simulink model "sschdlexSolarInverterSingleNetworkExample"  (R2023b)
settings: Solver=ode23t  StartTime=0.0  StopTime=.5  MaxStep=1e-4  RelTol=1e-3
PreLoadFcn:
  | load('EmulatedPV_LowPowerData.mat');
  | irr = 0.15;
  | numIrr = 10;
  | ArrayPower = ArrayCurrent.*ArrayVoltage;
  | 
  | C_Boost_In = 680e-6;
  | C_Boost_In_R = 0;
  | L_Boost = 100e-6;
  | L_Boost_R = 0;
  | C_Boost_Out = 1640e-6;
  | 
  | TsFPGA = 2e-6;
  | TsControl = 2e-6;
  | TsCPU = 2e-6;
  | Tc = TsControl;
  | Ts = 2e-6;
  | 
  | IGBT_Vth = 6;
  | IGBT_Vf = 0.8;
  | IGBT_R = 0.001;
  | IGBT_Con = 1e-5;
  | 
  | IGBT_D_Vth = 0.8;
  | IGBT_D_R = 0.001;
  | IGBT_D_Con = 1e-5;
  | 
  | maxIn = 10;
  | minIn = -10;
  | maxOut = 2^15;
  | minOut = -2^15;
  | difIn = maxIn-minIn;
  | difOut = maxOut-minOut;
  | gain = difOut/difIn;
  | dc1 = (maxOut+minOut)/2;
  | dc2 = (maxIn+minIn)/2;
  | offset = dc1-gain*dc2;
  | numIrr = 10;
  | ArrayPower = ArrayCurrent.*ArrayVoltage;
InitFcn:
  | Ts = 2e-6;
  | Tc = Ts;
values from neighbouring files (symbols this model uses):
  ArrayCurrent = [3 2.90135967378 2.78442846347 2.64406556825 2.47269969012 2.25842875672 1.98100825201 1.60223040661 1.04533074246 0.222841716608 0 0 ... (1000 elements, 100x10)]    [EmulatedPV_LowPowerData.mat]
  ArrayVoltage = [0 0.151515151515 0.30303030303 0.454545454545 0.606060606061 0.757575757576 0.909090909091 1.06060606061 1.21212121212 1.36363636364 1.51515151515 1.66666666667 ... (100 elements, 100x1)]    [EmulatedPV_LowPowerData.mat]
  Irradiance = [0.05 0.1 0.15 0.2 0.25 0.3 0.35 0.4 0.45 0.5]    [EmulatedPV_LowPowerData.mat]
undefined symbols (not defined in the file or in its folder): DiscIntNeverNeededParam, Tdata
libraries: fl_lib x20, nesl_utility x12, ee_lib x5, powerlib_meascontrol x4, simulink x3, slpidlib x2
CloseFcn:
  | clear ArrayCurrent
  | clear ArrayVoltage
  | clear Irradiance
  | 
  | clear irr;
  | clear numIrr;
  | clear ArrayPower;
  | 
  | clear C_Boost_In;
  | clear C_Boost_In_R;
  | clear L_Boost;
  | clear L_Boost_R;
  | clear C_Boost_Out;
  | 
  | clear TsFPGA;
  | clear TsControl;
  | clear TsCPU;
  | clear Tc;
  | clear Ts;
  | 
  | clear IGBT_Vth;
  | clear IGBT_Vf;
  | clear IGBT_R ;
  | clear IGBT_Con;
  | 
  | clear IGBT_D_Vth;
  | clear IGBT_D_R;
  | clear IGBT_D_Con;
  | 
  | clear maxIn;
  | clear minIn;
  | clear maxOut;
  | clear minOut;
  | clear difIn;
  | clear difOut;
  | clear gain;
  | clear dc1;
  | clear dc2;
  | clear offset;
settings Model: Creator=The MathWorks, Inc.  LastModifiedBy=The MathWorks, Inc.
settings SolverCC: AlgebraicLoopSolver=TrustRegion  AutoInsertRateTranBlk=on
settings OptimizationCC: BlockReduction=off  ConditionallyExecuteInputs=off  DefaultParameterBehavior=Inlined  EfficientMapNaN2IntZero=off
settings DebuggingCC: AlgebraicLoopMsg=error  SingleTaskRateTransMsg=error  ParameterPrecisionLossMsg=none  UnconnectedInputMsg=warning  UnconnectedOutputMsg=warning  UnconnectedLineMsg=warning  PregeneratedLibrarySubsystemCodeDiagnostic=none  ArithmeticOperatorsInVariantConditions=warning
settings HardwareCC: ProdBitPerPointer=32  ProdBitPerSizeT=32  ProdBitPerPtrDiffT=32  ProdLargestAtomicFloat=None  ProdIntDivRoundTo=Undefined  ProdEndianess=Unspecified  ProdWordSize=32  ProdHWDeviceType=ASIC/FPGA->ASIC/FPGA  TargetBitPerPointer=64  TargetBitPerSizeT=64  TargetBitPerPtrDiffT=64  TargetLongLongMode=on  TargetIntDivRoundTo=Zero  TargetEndianess=LittleEndian  TargetWordSize=64  TargetHWDeviceType=Custom Processor->MATLAB Host Computer  ProdEqTarget=off
settings ModelReferenceCC: EnableRefExpFcnMdlSchedulingChecks=on
settings SFSimCC: SimUseLocalCustomCode=off
settings CodeAppCC: MaxIdLength=128
settings GRTTargetCC: TargetLangStandard=C89/C90 (ANSI)  CombineOutputUpdateFcns=off  GRTInterface=on

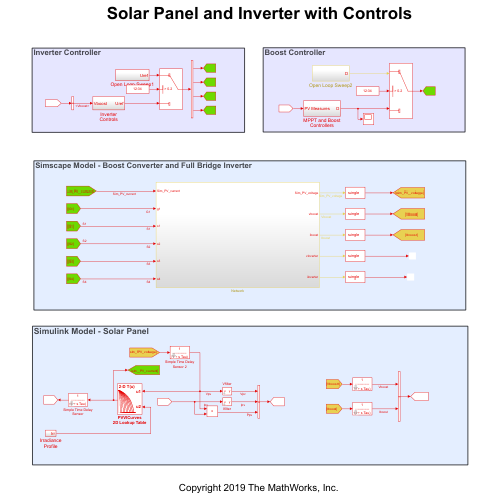
[thumbnail: Simulink's stored preview of the top-level diagram]
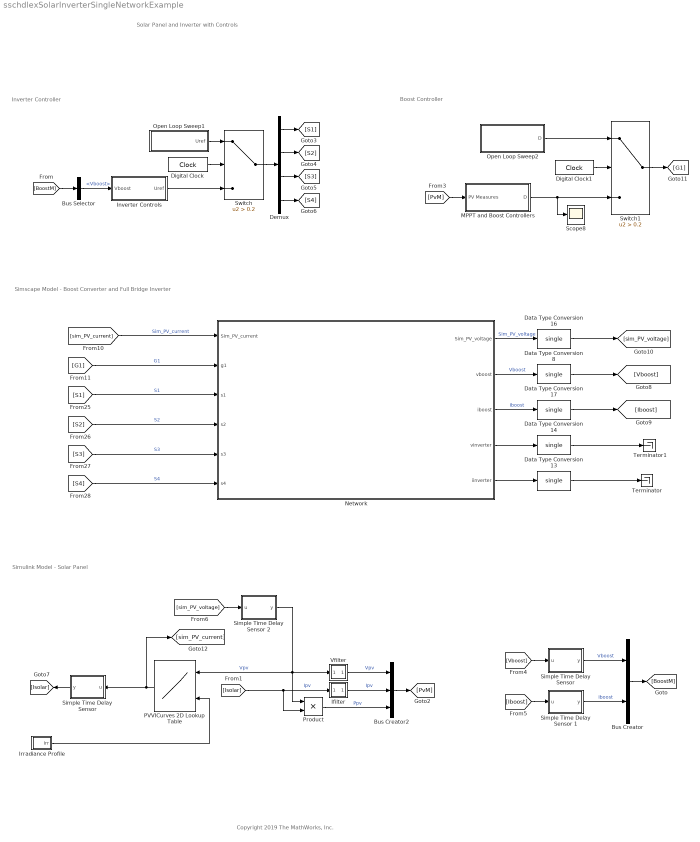
== system sschdlexSolarInverterSingleNetworkExample ==
  note: Solar Panel and Inverter with Controls
  note: Simulink Model - Solar Panel
  note: Inverter Controller
  note: Boost Controller
  note: Simscape Model - Boost Converter and Full Bridge Inverter
  note: Copyright 2019 The MathWorks, Inc.
  Bus Creator : BusCreator  Inputs=2
  Bus Creator2 : BusCreator  Inputs=3
  Bus Selector : BusSelector  OutputSignals=Vboost
  Data Type Conversion{13..14,16..17} (4 alike) : DataTypeConversion  OutDataTypeStr=single  RndMeth=Nearest  SaturateOnIntegerOverflow=off
  Data Type Conversion8 : DataTypeConversion  OutDataTypeStr=single  SaturateOnIntegerOverflow=off  RndMeth=Floor
  Demux : Demux
  Digital Clock : DigitalClock  SampleTime=2e-6
  Digital Clock1 : DigitalClock  SampleTime=2e-6
  Ifilter : Subsystem  mask{Tf=0.01}
      mask prompts: Tf "Filter Time Constant"
  Inverter Controls : Subsystem
  Irradiance Profile : Subsystem
  MPPT and Boost Controllers : Subsystem
  Network : Subsystem
  Open Loop Sweep1 : Subsystem
  Open Loop Sweep2 : Subsystem
  PVVICurves 2D Lookup Table : Lookup_n-D  BreakpointsForDimension1=ArrayVoltage  BreakpointsForDimension2=Irradiance  Table=ArrayCurrent  InternalRulePriority=Speed  RndMeth=Simplest
      settings: InputPortMap=u0,u1
  Product : Product
  Scope8 : Scope
  Simple Time Delay Sensor : Subsystem  mask{Ts=Ts, Tau=0.0001}
      mask prompts: Ts "Sample Time, [s]"; Tau "Time Constant, Tau [s]"
      mask help: Simple Sensor
      mask Display: fprintf('1\n------------\n(1 + s Tau)');
  "Simple Time Delay Sensor " : Subsystem  mask{Ts=Ts, Tau=0.0001}
      mask prompts: Ts "Sample Time, [s]"; Tau "Time Constant, Tau [s]"
      mask help: Simple Sensor
      mask Display: fprintf('1\n------------\n(1 + s Tau)');
  Simple Time Delay Sensor 1 : Subsystem  mask{Ts=Ts, Tau=0.0001}
      mask prompts: Ts "Sample Time, [s]"; Tau "Time Constant, Tau [s]"
      mask help: Simple Sensor
      mask Display: fprintf('1\n------------\n(1 + s Tau)');
  Simple Time Delay Sensor 2 : Subsystem  mask{Ts=Ts, Tau=0.0001}
      mask prompts: Ts "Sample Time, [s]"; Tau "Time Constant, Tau [s]"
      mask help: Simple Sensor
      mask Display: fprintf('1\n------------\n(1 + s Tau)');
  Switch : Switch  Criteria=u2 > Threshold  Threshold=0.2  SaturateOnIntegerOverflow=off  InputSameDT=off
  Switch1 : Switch  Criteria=u2 > Threshold  Threshold=0.2  SaturateOnIntegerOverflow=off  InputSameDT=off
  Terminator : Terminator
  Terminator1 : Terminator
  Vfilter : Subsystem  mask{Tf=0.01}
      mask prompts: Tf "Filter Time Constant"
  wires:
  Bus Creator/1 -> [BoostM]
  Demux/3 -> [S3]
  Demux/2 -> [S2]
  Irradiance Profile/1(Irr) -> PVVICurves 2D Lookup Table/2
  Product/1 -> Bus Creator2/3  "Ppv"
  Vfilter/1(y) -> Bus Creator2/1  "Vpv"
  [PvM] -> MPPT and Boost Controllers/1(PV Measures)
  PVVICurves 2D Lookup Table/1 -> Simple Time Delay Sensor/1(u), [sim_PV_current]
  [sim_PV_voltage] -> Simple Time Delay Sensor 2/1(u)
  MPPT and Boost Controllers/1(D) -> Scope8/1, Switch1/3
  [Iboost] -> Simple Time Delay Sensor 1/1(u)
  Open Loop Sweep1/1(Uref) -> Switch/1
  Bus Selector/1 -> Inverter Controls/1(Vboost)  "<Vboost>"
  Digital Clock1/1 -> Switch1/2
  Ifilter/1(y) -> Bus Creator2/2  "Ipv"
  [Isolar] -> Product/2, Ifilter/1(u)  "Ipv"
  Switch/1 -> Demux/1
  Switch1/1 -> [G1]
  Simple Time Delay Sensor/1(y) -> [Isolar]
  Bus Creator2/1 -> [PvM]
  Simple Time Delay Sensor 2/1(y) -> PVVICurves 2D Lookup Table/1, Product/1, Vfilter/1(u)  "Vpv"
  Simple Time Delay Sensor 1/1(y) -> Bus Creator/2  "Iboost"
  [Vboost] -> "Simple Time Delay Sensor "/1(u)
  Demux/1 -> [S1]
  Demux/4 -> [S4]
  [BoostM] -> Bus Selector/1
  Open Loop Sweep2/1(D) -> Switch1/1
  "Simple Time Delay Sensor "/1(y) -> Bus Creator/1  "Vboost"
  Inverter Controls/1(Uref) -> Switch/3
  Digital Clock/1 -> Switch/2
  [S4] -> Network/6(s4)  "S4"
  [S2] -> Network/4(s2)  "S2"
  [S1] -> Network/3(s1)  "S1"
  Data Type Conversion8/1 -> [Vboost]
  Data Type Conversion16/1 -> [sim_PV_voltage]
  Data Type Conversion17/1 -> [Iboost]
  [sim_PV_current] -> Network/1(Sim_PV_current)  "Sim_PV_current"
  Network/1(Sim_PV_voltage) -> Data Type Conversion16/1  "Sim_PV_voltage"
  Network/3(iboost) -> Data Type Conversion17/1  "Iboost"
  Network/2(vboost) -> Data Type Conversion8/1  "Vboost"
  [G1] -> Network/2(g1)  "G1"
  Data Type Conversion13/1 -> Terminator/1
  Data Type Conversion14/1 -> Terminator1/1
  [S3] -> Network/5(s3)  "S3"
  Network/4(vinverter) -> Data Type Conversion14/1
  Network/5(iinverter) -> Data Type Conversion13/1

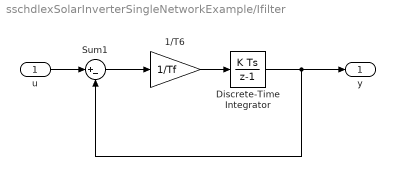
== system sschdlexSolarInverterSingleNetworkExample/Ifilter ==
  u : Inport
  1/T6 : Gain  Gain=1/Tf
  Discrete-Time Integrator : DiscreteIntegrator  SampleTime=Tc  ICPrevOutput=DiscIntNeverNeededParam  ICPrevScaledInput=DiscIntNeverNeededParam
  Sum1 : Sum  Inputs=|+-
  y : Outport  VectorParamsAs1DForOutWhenUnconnected=off
  wires:
  Sum1/1 -> 1/T6/1
  Discrete-Time Integrator/1 -> Sum1/2, y/1
  u/1 -> Sum1/1
  1/T6/1 -> Discrete-Time Integrator/1

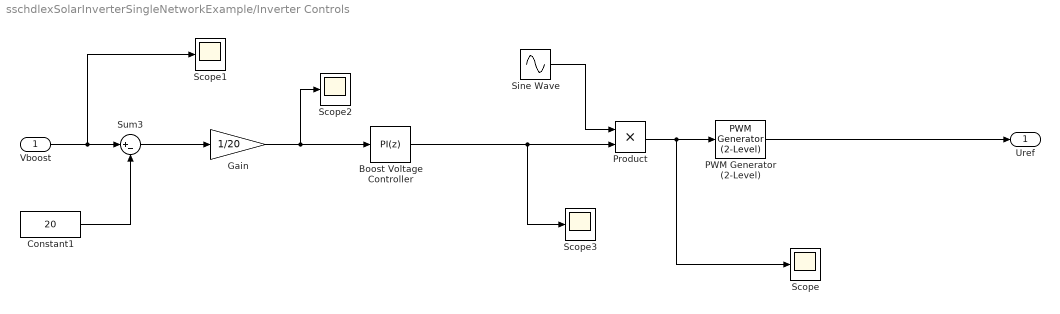
== system sschdlexSolarInverterSingleNetworkExample/Inverter Controls ==
  Vboost : Inport
  Boost Voltage Controller : slpidlib/PID Controller  Controller=PI  Form=Parallel  TimeDomain=Discrete-time  UseExternalTs=off  SampleTime=Tc  IntegratorMethod=Forward Euler  FilterMethod=Forward Euler  ControllerParametersSource=internal  P=4  I=500  UseKiTs=off  D=0  N=100  UseFilter=on  TunerSelectOption=Transfer Function Based (PID Tuner App)  InitialConditionSource=internal  InitialConditionForIntegrator=1  InitialConditionForFilter=0  DifferentiatorICPrevScaledInput=0  ExternalReset=none  TrackingMode=off  Kt=1  LimitOutput=on  SatLimitsSource=internal  UpperSaturationLimit=1  LowerSaturationLimit=0  LinearizeAsGain=on  AntiWindupMode=clamping  Kb=1  LimitIntegrator=off  UpperIntegratorSaturationLimit=inf  LowerIntegratorSaturationLimit=-inf  POutMin=[]  POutMax=[]  IOutMin=[]  IOutMax=[]  DOutMin=[]  DOutMax=[]  NOutMin=[]  NOutMax=[]  SumOutMin=[]  SumOutMax=[]  SaturationOutMin=[]  SaturationOutMax=[]  PParamMin=[]  PParamMax=[]  IParamMin=[]  IParamMax=[]  DParamMin=[]  DParamMax=[]  NParamMin=[]  NParamMax=[]  KbParamMin=[]  KbParamMax=[]  KtParamMin=[]  KtParamMax=[]  KbOutMin=[]  KbOutMax=[]  KtOutMin=[]  KtOutMax=[]  IntegratorOutMin=[]  IntegratorOutMax=[]  FilterOutMin=[]  FilterOutMax=[]  SumI1OutMin=[]  SumI1OutMax=[]  SumI2OutMin=[]  SumI2OutMax=[]  SumI3OutMin=[]  SumI3OutMax=[]  SumI4OutMin=[]  SumI4OutMax=[]  SumDOutMin=[]  SumDOutMax=[]  DifferentiatorOutMin=[]  DifferentiatorOutMax=[]  FilterDiffOutCoefMin=[]  FilterDiffOutCoefMax=[]  ReciprocalOutMin=[]  ReciprocalOutMax=[]  SumDenOutMin=[]  SumDenOutMax=[]  SumNumOutMin=[]  SumNumOutMax=[]  DivideOutMin=[]  DivideOutMax=[]  UdiffTsProdOutMin=[]  UdiffTsProdOutMax=[]  NTsProdOutMin=[]  NTsProdOutMax=[]  UintegralTsProdOutMin=[]  UintegralTsProdOutMax=[]  UngainTsProdOutMin=[]  UngainTsProdOutMax=[]  ClampingZeroOutDataTypeStr=Inherit: Inherit via back propagation  ClampingZeroOutMin=[]  ClampingZeroOutMax=[]  FilterDenConstantOutDataTypeStr=Inherit: Inherit via back propagation  FilterDenConstantOutMin=[]  FilterDenConstantOutMax=[]  PCopyOutDataTypeStr=Inherit: Inherit via back propagation  PCopyOutMin=[]  PCopyOutMax=[]  NCopyOutDataTypeStr=Inherit: Inherit via back propagation  NCopyOutMin=[]  NCopyOutMax=[]  IntegratorContinuousStateAttributes=''  IntegratorStateMustResolveToSignalObject=off  IntegratorRTWStateStorageClass=Auto  FilterContinuousStateAttributes=''  FilterStateMustResolveToSignalObject=off  FilterRTWStateStorageClass=Auto  ParallelPVariant=InternalParameters  IdealPVariant=Disabled  IVariant=InternalParameters  DVariant=Disabled  IntegratorVariant=Discrete  SatVariant=Enabled  AWVariant=DiscClampingParallel  PCopyVariant=Disabled  TRVariant=Disabled  FdbkBlocksVariant=Forward  IdealPFdbkVariant=Disabled  SatFdbkVariant=Disabled  DerivativeFilterVariant=Disabled  NVariant=Disabled  NCopyVariant=Disabled_SignalSpec  FilterICVariant=Disabled  IntegratorICVariant=InternalICs  ExternalResetVariant=Disabled  TRSumVariant=Passthrough  SumFdbkVariant=Disabled  SumVariant=Sum_PI  TsampFilterVariant=InternalTs  TsampNgainVariant=Passthrough  TsampIntegralVariant=Disabled_SignalSpec  ExternalSaturationOutDataTypeStr=Inherit: Same as second input
  Constant1 : Constant  Value=20
  Gain : Gain  Gain=1/20
  "PWM Generator (2-Level) " : powerlib_meascontrol/Pulse & Signal Generators/PWM Generator (2-Level)  ModulatorType=Single-phase full-bridge (4 pulses)  ModulatorMode=Unsynchronized  Fc=2000  Pc=90  nF=27  MinMax="[ -1  1 ]"  SamplingTechnique=Natural  ModulatingSignals=off  m=0.8  Freq=60  Phase=0  Ts=TsFPGA  ShowCarrierOutport=off
  Product : Product
  Scope{,1..3} (4 alike) : Scope
  Sine Wave : Sin  Frequency=2*pi*60  SampleTime=Tc
  Sum3 : Sum  Inputs=|+-
  Uref : Outport  VectorParamsAs1DForOutWhenUnconnected=off
  wires:
  Constant1/1 -> Sum3/2
  Sine Wave/1 -> Product/1
  Boost Voltage Controller/1 -> Scope3/1, Product/2
  Sum3/1 -> Gain/1
  Vboost/1 -> Scope1/1, Sum3/1
  Gain/1 -> Scope2/1, Boost Voltage Controller/1
  Product/1 -> Scope/1, "PWM Generator (2-Level) "/1
  "PWM Generator (2-Level) "/1 -> Uref/1

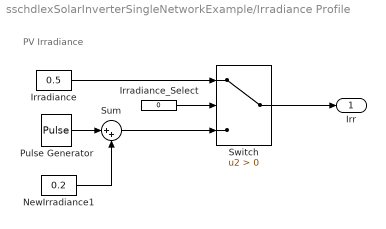
== system sschdlexSolarInverterSingleNetworkExample/Irradiance Profile ==
  note: PV Irradiance
  Irradiance : Constant  Value=0.5  OutDataTypeStr=single  SampleTime=2e-6
  Irradiance_Select : Constant  Value=0  OutDataTypeStr=single  SampleTime=2e-6
  NewIrradiance1 : Constant  Value=0.2  OutDataTypeStr=single  SampleTime=2e-6
  Pulse Generator : DiscretePulseGenerator  Amplitude=0.2  SampleTime=2e-6
  Sum : Sum  Inputs=|++
  Switch : Switch  Criteria=u2 > Threshold  SaturateOnIntegerOverflow=off  InputSameDT=off
  Irr : Outport  VectorParamsAs1DForOutWhenUnconnected=off
  wires:
  NewIrradiance1/1 -> Sum/2
  Pulse Generator/1 -> Sum/1
  Sum/1 -> Switch/3
  Irradiance/1 -> Switch/1
  Switch/1 -> Irr/1
  Irradiance_Select/1 -> Switch/2

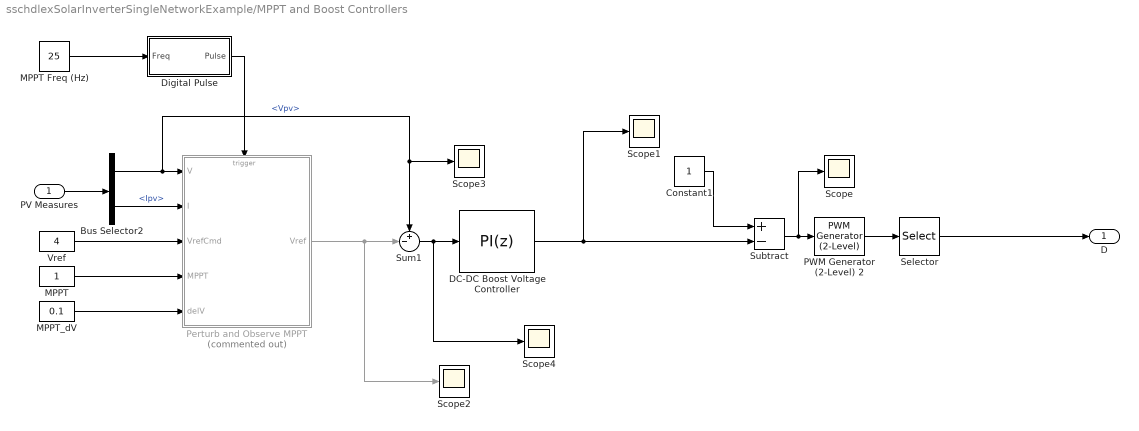
== system sschdlexSolarInverterSingleNetworkExample/MPPT and Boost Controllers ==
  PV Measures : Inport
  Bus Selector2 : BusSelector  OutputSignals=Vpv,Ipv
  Constant1 : Constant
  DC-DC Boost Voltage Controller : slpidlib/PID Controller  Controller=PI  Form=Parallel  TimeDomain=Discrete-time  UseExternalTs=off  SampleTime=Tc  IntegratorMethod=Forward Euler  FilterMethod=Forward Euler  ControllerParametersSource=internal  P=0.015  I=2.5  UseKiTs=off  D=0  N=100  UseFilter=on  TunerSelectOption=Transfer Function Based (PID Tuner App)  InitialConditionSource=internal  InitialConditionForIntegrator=0  InitialConditionForFilter=0  DifferentiatorICPrevScaledInput=0  ExternalReset=none  TrackingMode=off  Kt=1  LimitOutput=off  SatLimitsSource=internal  UpperSaturationLimit=0.9  LowerSaturationLimit=0  LinearizeAsGain=on  AntiWindupMode=clamping  Kb=1  LimitIntegrator=off  UpperIntegratorSaturationLimit=inf  LowerIntegratorSaturationLimit=-inf  POutMin=[]  POutMax=[]  IOutMin=[]  IOutMax=[]  DOutMin=[]  DOutMax=[]  NOutMin=[]  NOutMax=[]  SumOutMin=[]  SumOutMax=[]  SaturationOutMin=[]  SaturationOutMax=[]  PParamMin=[]  PParamMax=[]  IParamMin=[]  IParamMax=[]  DParamMin=[]  DParamMax=[]  NParamMin=[]  NParamMax=[]  KbParamMin=[]  KbParamMax=[]  KtParamMin=[]  KtParamMax=[]  KbOutMin=[]  KbOutMax=[]  KtOutMin=[]  KtOutMax=[]  IntegratorOutMin=[]  IntegratorOutMax=[]  FilterOutMin=[]  FilterOutMax=[]  SumI1OutMin=[]  SumI1OutMax=[]  SumI2OutMin=[]  SumI2OutMax=[]  SumI3OutMin=[]  SumI3OutMax=[]  SumI4OutMin=[]  SumI4OutMax=[]  SumDOutMin=[]  SumDOutMax=[]  DifferentiatorOutMin=[]  DifferentiatorOutMax=[]  FilterDiffOutCoefMin=[]  FilterDiffOutCoefMax=[]  ReciprocalOutMin=[]  ReciprocalOutMax=[]  SumDenOutMin=[]  SumDenOutMax=[]  SumNumOutMin=[]  SumNumOutMax=[]  DivideOutMin=[]  DivideOutMax=[]  UdiffTsProdOutMin=[]  UdiffTsProdOutMax=[]  NTsProdOutMin=[]  NTsProdOutMax=[]  UintegralTsProdOutMin=[]  UintegralTsProdOutMax=[]  UngainTsProdOutMin=[]  UngainTsProdOutMax=[]  ClampingZeroOutDataTypeStr=Inherit: Inherit via back propagation  ClampingZeroOutMin=[]  ClampingZeroOutMax=[]  FilterDenConstantOutDataTypeStr=Inherit: Inherit via back propagation  FilterDenConstantOutMin=[]  FilterDenConstantOutMax=[]  PCopyOutDataTypeStr=Inherit: Inherit via back propagation  PCopyOutMin=[]  PCopyOutMax=[]  NCopyOutDataTypeStr=Inherit: Inherit via back propagation  NCopyOutMin=[]  NCopyOutMax=[]  IntegratorContinuousStateAttributes=''  IntegratorStateMustResolveToSignalObject=off  IntegratorRTWStateStorageClass=Auto  FilterContinuousStateAttributes=''  FilterStateMustResolveToSignalObject=off  FilterRTWStateStorageClass=Auto  ParallelPVariant=InternalParameters  IdealPVariant=Disabled  IVariant=InternalParameters  DVariant=Disabled  IntegratorVariant=Discrete  SatVariant=Disabled  AWVariant=Passthrough  PCopyVariant=Disabled  TRVariant=Disabled  FdbkBlocksVariant=Forward  IdealPFdbkVariant=Disabled  SatFdbkVariant=Disabled  DerivativeFilterVariant=Disabled  NVariant=Disabled  NCopyVariant=Disabled_SignalSpec  FilterICVariant=Disabled  IntegratorICVariant=InternalICs  ExternalResetVariant=Disabled  TRSumVariant=Passthrough  SumFdbkVariant=Disabled  SumVariant=Sum_PI  TsampFilterVariant=InternalTs  TsampNgainVariant=Passthrough  TsampIntegralVariant=Disabled_SignalSpec  ExternalSaturationOutDataTypeStr=Inherit: Same as second input
  Digital Pulse : Subsystem  mask{Ts=Tc, Duty=0.5}
      mask prompts: Ts "Sample Rate [s]"; Duty "Duty Cycle [0-1]"
  MPPT : Constant
  MPPT Freq (Hz) : Constant  Value=25
  MPPT_dV : Constant  Value=0.1
  PWM Generator (2-Level) 2 : powerlib_meascontrol/Pulse & Signal Generators/PWM Generator (2-Level)  ModulatorType=Single-phase full-bridge (4 pulses)  ModulatorMode=Unsynchronized  Fc=2000  Pc=90  nF=27  MinMax=[0 1 ]  SamplingTechnique=Natural  ModulatingSignals=off  m=0.8  Freq=60  Phase=0  Ts=TsFPGA  ShowCarrierOutport=off
  Perturb and Observe MPPT : Subsystem  Commented=on  TreatAsAtomicUnit=on  SystemSampleTime=Tdata
  Scope{,1..4} (5 alike) : Scope
  Selector : Selector  InputPortWidth=4  IndexOptions=Index vector (dialog)  Indices=2  OutputSizes=1
  Subtract : Sum  Inputs=+-
  Sum1 : Sum  Inputs=+-|
  Vref : Constant  Value=4
  D : Outport  VectorParamsAs1DForOutWhenUnconnected=off
  wires:
  PV Measures/1 -> Bus Selector2/1
  Digital Pulse/1(Pulse) -> Perturb and Observe MPPT/Trigger
  MPPT Freq (Hz)/1 -> Digital Pulse/1(Freq)
  MPPT_dV/1 -> Perturb and Observe MPPT/5(delV)
  Vref/1 -> Perturb and Observe MPPT/3(VrefCmd)
  Sum1/1 -> Scope4/1, DC-DC Boost Voltage Controller/1
  MPPT/1 -> Perturb and Observe MPPT/4(MPPT)
  Bus Selector2/1 -> Perturb and Observe MPPT/1(V), Scope3/1, Sum1/1  "<Vpv>"
  Perturb and Observe MPPT/1(Vref) -> Scope2/1, Sum1/2
  Bus Selector2/2 -> Perturb and Observe MPPT/2(I)  "<Ipv>"
  Selector/1 -> D/1
  PWM Generator (2-Level) 2/1 -> Selector/1
  Constant1/1 -> Subtract/1
  DC-DC Boost Voltage Controller/1 -> Scope1/1, Subtract/2
  Subtract/1 -> Scope/1, PWM Generator (2-Level) 2/1

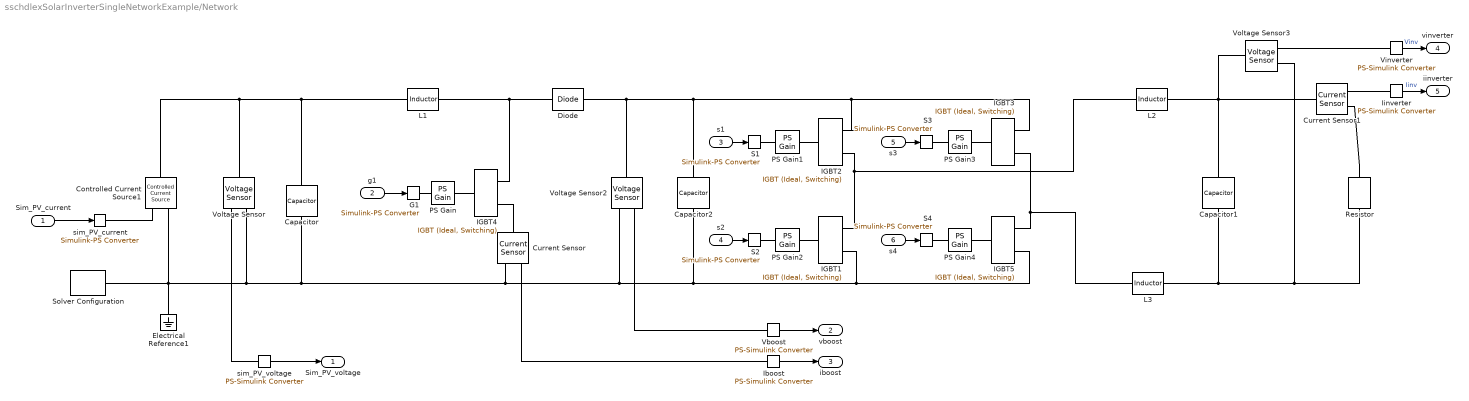
== system sschdlexSolarInverterSingleNetworkExample/Network ==
  Sim_PV_current : Inport
  g1 : Inport  Port=2
  s1 : Inport  Port=3
  s2 : Inport  Port=4
  s3 : Inport  Port=5
  s4 : Inport  Port=6
  Capacitor : fl_lib/Electrical/Electrical Elements/Capacitor  c=C_Boost_In F  r=C_Boost_In_R Ohm  g=0 1/Ohm  i_specify=off  i_priority=None  i=0 A  i_nominal_specify=off  i_nominal_unit=A  i_nominal_value=1  v_specify=off  v_priority=None  v=0 V  v_nominal_specify=off  v_nominal_unit=V  v_nominal_value=1  vc_specify=off  vc_priority=High  vc=0 V  vc_nominal_specify=off  vc_nominal_unit=V  vc_nominal_value=1
  Capacitor1 : fl_lib/Electrical/Electrical Elements/Capacitor  c=3e-6 F  r=0 Ohm  g=0 1/Ohm  i_specify=off  i_priority=None  i=0 A  i_nominal_specify=off  i_nominal_unit=A  i_nominal_value=1  v_specify=off  v_priority=None  v=0 V  v_nominal_specify=off  v_nominal_unit=V  v_nominal_value=1  vc_specify=off  vc_priority=High  vc=0 V  vc_nominal_specify=off  vc_nominal_unit=V  vc_nominal_value=1
  Capacitor2 : fl_lib/Electrical/Electrical Elements/Capacitor  c=2*1640e-6 F  r=0.0005 Ohm  g=0 1/Ohm  i_specify=off  i_priority=None  i=0 A  i_nominal_specify=off  i_nominal_unit=A  i_nominal_value=1  v_specify=off  v_priority=None  v=0 V  v_nominal_specify=off  v_nominal_unit=V  v_nominal_value=1  vc_specify=off  vc_priority=High  vc=0 V  vc_nominal_specify=off  vc_nominal_unit=V  vc_nominal_value=1
  Controlled Current Source1 : fl_lib/Electrical/Electrical Sources/Controlled Current Source
  Current Sensor : fl_lib/Electrical/Electrical Sensors/Current Sensor
  Current Sensor1 : fl_lib/Electrical/Electrical Sensors/Current Sensor
  Diode : fl_lib/Electrical/Electrical Elements/Diode  Vf=0.8 V  Ron=0.001 Ohm  Goff=1e-8 1/Ohm  i_specify=off  i_priority=None  i=0 A  i_nominal_specify=off  i_nominal_unit=A  i_nominal_value=1  v_specify=off  v_priority=None  v=0 V  v_nominal_specify=off  v_nominal_unit=V  v_nominal_value=1
  Electrical Reference1 : fl_lib/Electrical/Electrical Elements/Electrical Reference
  G1 : nesl_utility/Simulink-PS Converter  PhysicalDomain=network_engine_domain  SubClassName=ps_input  LeftPortType=input  RightPortType=output  PseudoPeriodic=off  Frequencies=[]  NoiseDistribution=none  NoiseParameters=[]  Unit=1  AffineConversion=off  FilteringAndDerivatives=provide  SimscapeFilterOrder=1  InputFilterTimeConstant=0.001  UdotUserProvided=0
  IGBT{1..5} (5 alike) : ee_lib/Semiconductors & Converters/IGBT (Ideal, Switching)  Vf=IGBT_Vf V  Ron=IGBT_R Ohm  Goff=IGBT_Con 1/Ohm  Vth=IGBT_Vth V  diode_param=2  diode_Vf=IGBT_D_Vth V  diode_Ron=IGBT_D_R Ohm  diode_Goff=IGBT_D_Con 1/Ohm  diode_C=5e-8 F  diode_iRM=-235 A  diode_iF=300 A  diode_idot=-50 A/us  diode_trr_param=1  diode_trr_factor=3  diode_trr=15 us  diode_Qrr=1.5e+3 s*uA  thermal_loss_option=2  Voff=300 V  Tau=1e-4 s  Tj=[298.15, 398.15] K  Iout_scalar=600 A  Eon_scalar=22.86e-3 J  Eoff_scalar=17.14e-3 J  Von_scalar=2.7 V  Iout_data=[0, 10, 50, 100, 200, 400, 600] A  Eon_data=[0, .29, 1.43, 2.86, 5.71, 13.14, 22.86; 0, .57, 2.63, 5.14, 10.29, 20.57, 30.29] * 1e-3 J  Eoff_data=[0, .21, 1.07, 2.14, 4.29, 9.86, 17.14; 0, .43, 1.97, 3.86, 7.71, 15.43, 22.71] * 1e-3 J  Von_data=[0, 1.1, 1.3, 1.45, 1.75, 2.25, 2.7; 0, 1, 1.15, 1.35, 1.7, 2.35, 3] V
  Iboost : nesl_utility/PS-Simulink Converter  PhysicalDomain=network_engine_domain  SubClassName=ps_output  LeftPortType=input  RightPortType=output  PseudoPeriodic=off  Frequencies=[]  Unit=1  AffineConversion=off
  Iinverter : nesl_utility/PS-Simulink Converter  PhysicalDomain=network_engine_domain  SubClassName=ps_output  LeftPortType=input  RightPortType=output  PseudoPeriodic=off  Frequencies=[]  Unit=1  AffineConversion=off
  L1 : fl_lib/Electrical/Electrical Elements/Inductor  l=L_Boost H  r=L_Boost_R Ohm  g=1e-9 1/Ohm  i_specify=off  i_priority=None  i=0 A  i_nominal_specify=off  i_nominal_unit=A  i_nominal_value=1  v_specify=off  v_priority=None  v=0 V  v_nominal_specify=off  v_nominal_unit=V  v_nominal_value=1  i_L_specify=off  i_L_priority=High  i_L=0 A  i_L_nominal_specify=off  i_L_nominal_unit=A  i_L_nominal_value=1
      settings: AttributesFormatString=|
      | %<l> H
      | %<r> Ohm
  L2 : fl_lib/Electrical/Electrical Elements/Inductor  l=100e-6 H  r=0.001 Ohm  g=1e-9 1/Ohm  i_specify=off  i_priority=None  i=0 A  i_nominal_specify=off  i_nominal_unit=A  i_nominal_value=1  v_specify=off  v_priority=None  v=0 V  v_nominal_specify=off  v_nominal_unit=V  v_nominal_value=1  i_L_specify=off  i_L_priority=High  i_L=0 A  i_L_nominal_specify=off  i_L_nominal_unit=A  i_L_nominal_value=1
      settings: AttributesFormatString=|
      | %<l> H
      | %<r> Ohm
  L3 : fl_lib/Electrical/Electrical Elements/Inductor  l=100e-6 H  r=0.001 Ohm  g=1e-9 1/Ohm  i_specify=off  i_priority=None  i=0 A  i_nominal_specify=off  i_nominal_unit=A  i_nominal_value=1  v_specify=off  v_priority=None  v=0 V  v_nominal_specify=off  v_nominal_unit=V  v_nominal_value=1  i_L_specify=off  i_L_priority=High  i_L=0 A  i_L_nominal_specify=off  i_L_nominal_unit=A  i_L_nominal_value=1
      settings: AttributesFormatString=|
      | %<l> H
      | %<r> Ohm
  PS Gain{,1..4} (5 alike) : fl_lib/Physical Signals/Functions/PS Gain  gain=1.5*IGBT_Vth
  Resistor : fl_lib/Electrical/Electrical Elements/Resistor  R=11.5 Ohm  i_specify=off  i_priority=None  i=0 A  i_nominal_specify=off  i_nominal_unit=A  i_nominal_value=1  v_specify=off  v_priority=None  v=0 V  v_nominal_specify=off  v_nominal_unit=V  v_nominal_value=1
  S{1..4} (4 alike) : nesl_utility/Simulink-PS Converter  PhysicalDomain=network_engine_domain  SubClassName=ps_input  LeftPortType=input  RightPortType=output  PseudoPeriodic=off  Frequencies=[]  NoiseDistribution=none  NoiseParameters=[]  Unit=1  AffineConversion=off  FilteringAndDerivatives=provide  SimscapeFilterOrder=1  InputFilterTimeConstant=0.001  UdotUserProvided=0
  Solver Configuration : nesl_utility/Solver Configuration  PhysicalDomain=network_engine_domain  SubClassName=solver  LeftPortType=input  RightPortType=generic  Tones=[]  Harmonics=[]  SimulateNoise=off  Profile=off  UseLocalSampling=off  EnableSwitchedLinearOptims=on  FrequencyDomain=off  UseCCode=off  RelTol=0.001  AbsTol=1e-06  MinStep=1e-09  ToWorkspace=off  RevertToSquareIcSolve=off  NumHomotopyIterations=100  PhasorMode=off  PhasorModeNumHarmonics=1  DoDC=off  ResidualTolerance=1e-09  UseLocalSolver=on  LocalSolverChoice=NE_BACKWARD_EULER_ADVANCER  LocalSolverSampleTime=2e-6  DoFixedCost=off  MaxNonlinIter=3  MaxModeIter=2  LinearAlgebra=auto  EquationFormulation=NE_TIME_EF  DelaysMemoryBudget=1024  AutomaticFiltering=on  FilteringTimeConstant=0.001  PartitionStorageMethod=AS_NEEDED  PartitionMemoryBudget=1024  PartitionMethod=FAST
  Vboost : nesl_utility/PS-Simulink Converter  PhysicalDomain=network_engine_domain  SubClassName=ps_output  LeftPortType=input  RightPortType=output  PseudoPeriodic=off  Frequencies=[]  Unit=1  AffineConversion=off
  Vinverter : nesl_utility/PS-Simulink Converter  PhysicalDomain=network_engine_domain  SubClassName=ps_output  LeftPortType=input  RightPortType=output  PseudoPeriodic=off  Frequencies=[]  Unit=1  AffineConversion=off
  Voltage Sensor : fl_lib/Electrical/Electrical Sensors/Voltage Sensor
  Voltage Sensor2 : fl_lib/Electrical/Electrical Sensors/Voltage Sensor
  Voltage Sensor3 : fl_lib/Electrical/Electrical Sensors/Voltage Sensor
  sim_PV_current : nesl_utility/Simulink-PS Converter  PhysicalDomain=network_engine_domain  SubClassName=ps_input  LeftPortType=input  RightPortType=output  PseudoPeriodic=off  Frequencies=[]  NoiseDistribution=none  NoiseParameters=[]  Unit=1  AffineConversion=off  FilteringAndDerivatives=provide  SimscapeFilterOrder=1  InputFilterTimeConstant=0.001  UdotUserProvided=0
  sim_PV_voltage : nesl_utility/PS-Simulink Converter  PhysicalDomain=network_engine_domain  SubClassName=ps_output  LeftPortType=input  RightPortType=output  PseudoPeriodic=off  Frequencies=[]  Unit=1  AffineConversion=off
  Sim_PV_voltage : Outport
  vboost : Outport  Port=2
  iboost : Outport  Port=3
  vinverter : Outport  Port=4
  iinverter : Outport  Port=5
  wires:
  s1/1 -> S1/1
  Iinverter/1 -> iinverter/1  "Iinv"
  Sim_PV_current/1 -> sim_PV_current/1
  g1/1 -> G1/1
  s4/1 -> S4/1
  s3/1 -> S3/1
  Vboost/1 -> vboost/1
  Iboost/1 -> iboost/1
  Vinverter/1 -> vinverter/1  "Vinv"
  s2/1 -> S2/1
  sim_PV_voltage/1 -> Sim_PV_voltage/1
  connections:
  Capacitor/RConn1 -- Controlled Current Source1/RConn2 -- Electrical Reference1/LConn1 -- Solver Configuration/RConn1 -- Voltage Sensor/RConn2 -- IGBT5/RConn2 -- IGBT1/RConn2 -- Capacitor2/RConn1 -- Voltage Sensor2/RConn2 -- Current Sensor/RConn2
  L1/RConn1 -- IGBT4/RConn1 -- Diode/LConn1
  Voltage Sensor3/RConn2 -- Resistor/RConn1 -- Capacitor1/RConn1 -- L3/RConn1
  Diode/RConn1 -- Voltage Sensor2/LConn1 -- IGBT3/RConn1 -- IGBT2/RConn1 -- Capacitor2/LConn1
  IGBT3/RConn2 -- L3/LConn1 -- IGBT5/RConn1
  L1/LConn1 -- Controlled Current Source1/LConn1 -- Voltage Sensor/LConn1 -- Capacitor/LConn1
  IGBT1/RConn1 -- L2/LConn1 -- IGBT2/RConn2
  Capacitor1/LConn1 -- Current Sensor1/LConn1 -- L2/RConn1 -- Voltage Sensor3/LConn1
  PS Gain4/LConn1 -- S4/RConn1
  PS Gain3/LConn1 -- S3/RConn1
  Current Sensor/RConn1 -- Iboost/LConn1
  Resistor/LConn1 -- Current Sensor1/RConn2
  PS Gain1/LConn1 -- S1/RConn1
  PS Gain2/LConn1 -- S2/RConn1
  Voltage Sensor2/RConn1 -- Vboost/LConn1
  IGBT1/LConn1 -- PS Gain2/RConn1
  IGBT3/LConn1 -- PS Gain3/RConn1
  PS Gain/RConn1 -- IGBT4/LConn1
  IGBT5/LConn1 -- PS Gain4/RConn1
  Iinverter/LConn1 -- Current Sensor1/RConn1
  Voltage Sensor3/RConn1 -- Vinverter/LConn1
  Controlled Current Source1/RConn1 -- sim_PV_current/RConn1
  sim_PV_voltage/LConn1 -- Voltage Sensor/RConn1
  G1/RConn1 -- PS Gain/LConn1
  IGBT2/LConn1 -- PS Gain1/RConn1
  IGBT4/RConn2 -- Current Sensor/LConn1

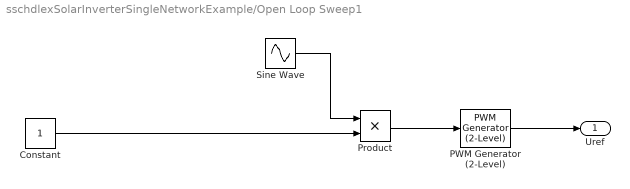
== system sschdlexSolarInverterSingleNetworkExample/Open Loop Sweep1 ==
  Constant : Constant
  "PWM Generator (2-Level) " : powerlib_meascontrol/Pulse & Signal Generators/PWM Generator (2-Level)  ModulatorType=Single-phase full-bridge (4 pulses)  ModulatorMode=Unsynchronized  Fc=2000  Pc=90  nF=27  MinMax="[ -1  1 ]"  SamplingTechnique=Natural  ModulatingSignals=off  m=0.8  Freq=60  Phase=0  Ts=TsFPGA  ShowCarrierOutport=off
  Product : Product
  Sine Wave : Sin  Amplitude=0.9  Frequency=2*pi*60*2  SampleTime=Tc
  Uref : Outport  VectorParamsAs1DForOutWhenUnconnected=off
  wires:
  "PWM Generator (2-Level) "/1 -> Uref/1
  Product/1 -> "PWM Generator (2-Level) "/1
  Constant/1 -> Product/2
  Sine Wave/1 -> Product/1

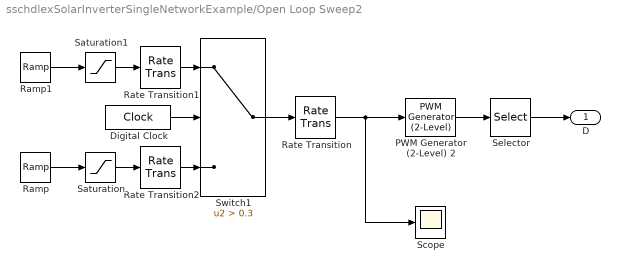
== system sschdlexSolarInverterSingleNetworkExample/Open Loop Sweep2 ==
  Digital Clock : DigitalClock  SampleTime=2e-6
  PWM Generator (2-Level) 2 : powerlib_meascontrol/Pulse & Signal Generators/PWM Generator (2-Level)  ModulatorType=Single-phase full-bridge (4 pulses)  ModulatorMode=Unsynchronized  Fc=2000  Pc=90  nF=27  MinMax=[0 1 ]  SamplingTechnique=Natural  ModulatingSignals=off  m=0.8  Freq=60  Phase=0  Ts=TsFPGA  ShowCarrierOutport=off
  Ramp : simulink/Sources/Ramp  slope=8  start=0.2  InitialOutput=0.1
  Ramp1 : simulink/Sources/Ramp  slope=8  start=0.3  InitialOutput=0.1
  Rate Transition : RateTransition  OutPortSampleTime=2e-6
  Rate Transition1 : RateTransition  OutPortSampleTime=2e-6
  Rate Transition2 : RateTransition  OutPortSampleTime=2e-6
  Saturation : Saturate  UpperLimit=1  LowerLimit=0
  Saturation1 : Saturate  UpperLimit=1  LowerLimit=0
  Scope : Scope
  Selector : Selector  InputPortWidth=4  IndexOptions=Index vector (dialog)  Indices=2  OutputSizes=1
  Switch1 : Switch  Criteria=u2 > Threshold  Threshold=0.3  SaturateOnIntegerOverflow=off  InputSameDT=off
  D : Outport  VectorParamsAs1DForOutWhenUnconnected=off
  wires:
  Ramp/1 -> Saturation/1
  Selector/1 -> D/1
  PWM Generator (2-Level) 2/1 -> Selector/1
  Switch1/1 -> Rate Transition/1
  Digital Clock/1 -> Switch1/2
  Ramp1/1 -> Saturation1/1
  Saturation1/1 -> Rate Transition1/1
  Saturation/1 -> Rate Transition2/1
  Rate Transition/1 -> Scope/1, PWM Generator (2-Level) 2/1
  Rate Transition2/1 -> Switch1/3
  Rate Transition1/1 -> Switch1/1

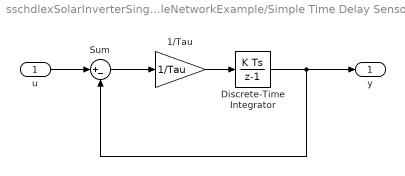
== system sschdlexSolarInverterSingleNetworkExample/Simple Time Delay Sensor ==
  u : Inport
  1/Tau : Gain  Gain=1/Tau
  Discrete-Time Integrator : DiscreteIntegrator  SampleTime=Ts  ICPrevOutput=DiscIntNeverNeededParam  ICPrevScaledInput=DiscIntNeverNeededParam
  Sum : Sum  Inputs=|+-
  y : Outport  VectorParamsAs1DForOutWhenUnconnected=off
  wires:
  1/Tau/1 -> Discrete-Time Integrator/1
  Sum/1 -> 1/Tau/1
  u/1 -> Sum/1
  Discrete-Time Integrator/1 -> y/1, Sum/2

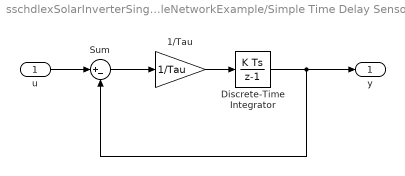
== system sschdlexSolarInverterSingleNetworkExample/Simple Time Delay Sensor  ==
  u : Inport
  1/Tau : Gain  Gain=1/Tau
  Discrete-Time Integrator : DiscreteIntegrator  SampleTime=Ts  ICPrevOutput=DiscIntNeverNeededParam  ICPrevScaledInput=DiscIntNeverNeededParam
  Sum : Sum  Inputs=|+-
  y : Outport  VectorParamsAs1DForOutWhenUnconnected=off
  wires:
  Discrete-Time Integrator/1 -> Sum/2, y/1
  u/1 -> Sum/1
  Sum/1 -> 1/Tau/1
  1/Tau/1 -> Discrete-Time Integrator/1

== system sschdlexSolarInverterSingleNetworkExample/Simple Time Delay Sensor 1 ==
  u : Inport
  1/Tau : Gain  Gain=1/Tau
  Discrete-Time Integrator : DiscreteIntegrator  SampleTime=Ts  ICPrevOutput=DiscIntNeverNeededParam  ICPrevScaledInput=DiscIntNeverNeededParam
  Sum : Sum  Inputs=|+-
  y : Outport  VectorParamsAs1DForOutWhenUnconnected=off
  wires:
  1/Tau/1 -> Discrete-Time Integrator/1
  Sum/1 -> 1/Tau/1
  u/1 -> Sum/1
  Discrete-Time Integrator/1 -> y/1, Sum/2

== system sschdlexSolarInverterSingleNetworkExample/Simple Time Delay Sensor 2 ==
  u : Inport
  1/Tau : Gain  Gain=1/Tau
  Discrete-Time Integrator : DiscreteIntegrator  SampleTime=Ts  ICPrevOutput=DiscIntNeverNeededParam  ICPrevScaledInput=DiscIntNeverNeededParam
  Sum : Sum  Inputs=|+-
  y : Outport  VectorParamsAs1DForOutWhenUnconnected=off
  wires:
  Discrete-Time Integrator/1 -> Sum/2, y/1
  u/1 -> Sum/1
  Sum/1 -> 1/Tau/1
  1/Tau/1 -> Discrete-Time Integrator/1

== system sschdlexSolarInverterSingleNetworkExample/Vfilter ==
  u : Inport
  1/T6 : Gain  Gain=1/Tf
  Discrete-Time Integrator : DiscreteIntegrator  SampleTime=Tc  ICPrevOutput=DiscIntNeverNeededParam  ICPrevScaledInput=DiscIntNeverNeededParam
  Sum1 : Sum  Inputs=|+-
  y : Outport  VectorParamsAs1DForOutWhenUnconnected=off
  wires:
  1/T6/1 -> Discrete-Time Integrator/1
  u/1 -> Sum1/1
  Discrete-Time Integrator/1 -> y/1, Sum1/2
  Sum1/1 -> 1/T6/1

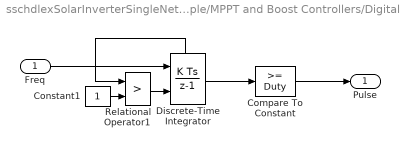
== system sschdlexSolarInverterSingleNetworkExample/MPPT and Boost Controllers/Digital Pulse ==
  Freq : Inport
  Compare To Constant : simulink/Logic and Bit Operations/Compare To Constant  relop=>=  const=Duty  OutDataTypeStr=boolean
  Constant1 : Constant
  Discrete-Time Integrator : DiscreteIntegrator  ExternalReset=rising  SampleTime=Ts  ShowStatePort=on  ICPrevOutput=DiscIntNeverNeededParam  ICPrevScaledInput=DiscIntNeverNeededParam
  Relational Operator1 : RelationalOperator  Operator=>  OutDataTypeStr=boolean  InputSameDT=off
  Pulse : Outport  VectorParamsAs1DForOutWhenUnconnected=off
  wires:
  Relational Operator1/1 -> Discrete-Time Integrator/2
  Constant1/1 -> Relational Operator1/2
  Compare To Constant/1 -> Pulse/1
  Discrete-Time Integrator/State -> Relational Operator1/1
  Discrete-Time Integrator/1 -> Compare To Constant/1
  Freq/1 -> Discrete-Time Integrator/1

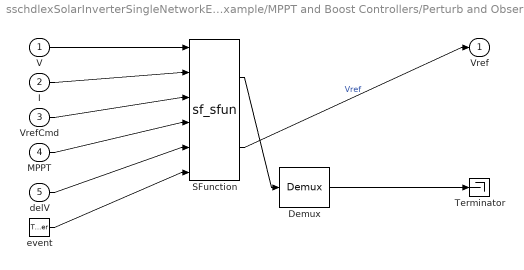
== system sschdlexSolarInverterSingleNetworkExample/MPPT and Boost Controllers/Perturb and Observe MPPT ==
  V : Inport
  I : Inport  Port=2
  VrefCmd : Inport  Port=3
  MPPT : Inport  Port=4
  delV : Inport  Port=5
  event : TriggerPort  VariantControl=(inherit)  ShowOutputPort=on
  " Demux " : Demux  Outputs=1
      settings: DisplayOption=none
  " SFunction " : S-Function  Tag=Stateflow S-Function 3  FunctionName=sf_sfun  PortCounts=[6 2]  SFunctionDeploymentMode=off  EnableBusSupport=on
  " Terminator " : Terminator
  Vref : Outport  VectorParamsAs1DForOutWhenUnconnected=off
  wires:
  V/1 -> " SFunction "/1
  I/1 -> " SFunction "/2
  VrefCmd/1 -> " SFunction "/3
  MPPT/1 -> " SFunction "/4
  delV/1 -> " SFunction "/5
  " SFunction "/2 -> Vref/1  "Vref"
  event/1 -> " SFunction "/6
  " Demux "/1 -> " Terminator "/1
  " SFunction "/1 -> " Demux "/1
